simulink model "RealTimeSimulation"  (R2024b)
settings: Solver=ode45  StartTime=0.0  StopTime=20  FixedStep=0.001  RelTol=1e-3
InitFcn:
  | Init
values from neighbouring files (symbols this model uses):
  Beq = 1.223604206496999e-06    (= 1.2236042065e-06)    [DesignPart567.m]    (also in DesignPart9Sine.m; DesignPart9Step.m; Init.m; Real_time_parameter_estimation.m = (data.Beq_hat_pos + data.Beq_hat_neg)/2)
  degs2rpm = 60/360    (= 0.166666666667)    [Init.m]
  delta_est = 1/sqrt(2)    [DesignPart9Step.m]    (also in Init.m)
  Kd = Kp * Td    [Init.m]
  Ki = Kp / Ti    [Init.m]
  Kp = deltak * cos(deltaphi)    [Init.m]
  rpm2degs = 360/60    (= 6)    [Init.m]
  rpm2rads = 2*pi/60    (= 0.10471975512)    [Init.m]
  tau_sf = (abs(data.tau_sf_pos)+abs(data.tau_sf_neg))/2    [Real_time_parameter_estimation.m]    (also in real-time-estimation.mat = 0.0046178193958)
  tl = 1/(3*wgc)    [Init.m]
  wc = 2*pi*50    (= 314.159265359)    [DesignPart9Step.m]    (also in Init.m; State_space_1324.m)
undefined symbols (not defined in the file or in its folder): gbox, mot, sens
libraries: simulink x2
settings Model: Creator=Banaan  LastModifiedBy=lucag

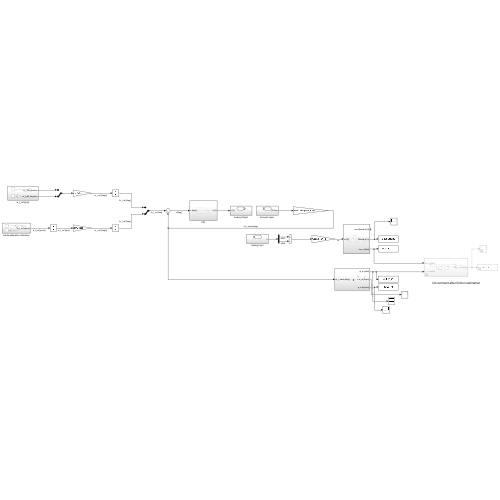
[thumbnail: Simulink's stored preview of the top-level diagram]
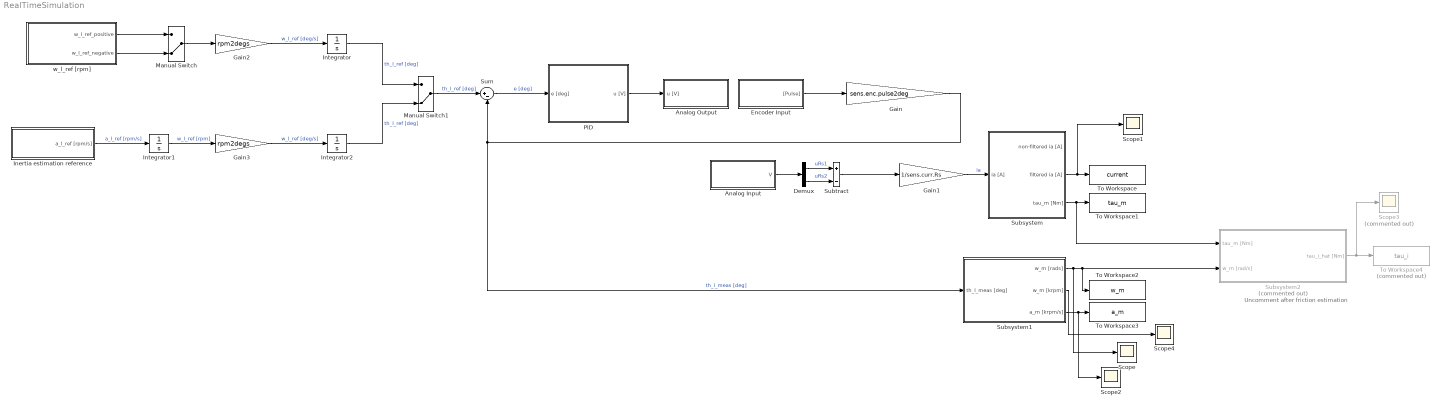
== system RealTimeSimulation ==
  note: Uncomment after friction estimation
  Analog Input : Subsystem
  Analog Output : Subsystem
  Demux : Demux  Outputs=2
  Encoder Input : Subsystem
  Gain : Gain  Gain=sens.enc.pulse2deg
  Gain1 : Gain  Gain=1/sens.curr.Rs
  Gain2 : Gain  Gain=rpm2degs
  Gain3 : Gain  Gain=rpm2degs
  Inertia estimation reference : Subsystem
  Integrator : Integrator
  Integrator1 : Integrator
  Integrator2 : Integrator
  Manual Switch : ManualSwitch  CurrentSetting=0
  Manual Switch1 : ManualSwitch  CurrentSetting=0
  PID : Subsystem
  Scope{,1..2,4} (4 alike) : Scope
  Scope3 : Scope  Commented=on
  Subsystem : Subsystem
  Subsystem1 : Subsystem
  Subsystem2 : Subsystem  Commented=on
  Subtract : Sum  Inputs=+-
  Sum : Sum  Inputs=|+-
  To Workspace : ToWorkspace  VariableName=current  SaveFormat=Structure With Time  SampleTime=-1
  To Workspace1 : ToWorkspace  VariableName=tau_m  SaveFormat=Structure With Time  SampleTime=-1
  To Workspace2 : ToWorkspace  VariableName=w_m  SaveFormat=Structure With Time  SampleTime=-1
  To Workspace3 : ToWorkspace  VariableName=a_m  SaveFormat=Structure With Time  SampleTime=-1
  To Workspace4 : ToWorkspace  Commented=on  VariableName=tau_i  SaveFormat=Structure With Time  SampleTime=-1
  w_l_ref [rpm] : Subsystem
  wires:
  Gain/1 -> Subsystem1/1(th_l_meas [deg]), Sum/2  "th_l_meas [deg]"
  Sum/1 -> PID/1(e [deg])  "e [deg]"
  Manual Switch1/1 -> Sum/1  "th_l_ref [deg]"
  Analog Input/1(V) -> Demux/1
  Demux/1 -> Subtract/1  "uRs1"
  Demux/2 -> Subtract/2  "uRs2"
  Gain1/1 -> Subsystem/1(ia [A])  "ia"
  Subsystem/2(filtered ia [A]) -> Scope1/1, To Workspace/1
  Subsystem/3(tau_m [Nm]) -> Subsystem2/1(tau_m [Nm]), To Workspace1/1
  Gain2/1 -> Integrator/1  "w_l_ref [deg/s]"
  Integrator/1 -> Manual Switch1/1  "th_l_ref [deg]"
  Gain3/1 -> Integrator2/1  "w_l_ref [deg/s]"
  Inertia estimation reference/1(a_l_ref [rpm/s]) -> Integrator1/1  "a_l_ref [rpm/s]"
  Integrator1/1 -> Gain3/1  "w_l_ref [rpm]"
  Integrator2/1 -> Manual Switch1/2  "th_l_ref [deg]"
  Manual Switch/1 -> Gain2/1
  w_l_ref [rpm]/1(w_l_ref_positive) -> Manual Switch/1
  w_l_ref [rpm]/2(w_l_ref_negative) -> Manual Switch/2
  Subsystem1/1(w_m [rads]) -> Subsystem2/2(w_m [rad/s]), To Workspace2/1, Scope/1
  Subsystem1/3(a_m [krpm/s]) -> Scope2/1, To Workspace3/1
  Subsystem2/1(tau_i_hat [Nm]) -> Scope3/1, To Workspace4/1
  Subsystem1/2(w_m [krpm]) -> Scope4/1
  PID/1(u [V]) -> Analog Output/1(u [V])
  Encoder Input/1("[Pulse]") -> Gain/1
  Subtract/1 -> Gain1/1

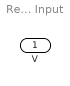
== system RealTimeSimulation/Analog Input ==
  V : Outport

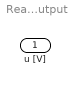
== system RealTimeSimulation/Analog Output ==
  u [V] : Inport

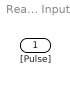
== system RealTimeSimulation/Encoder Input ==
  "[Pulse]" : Outport

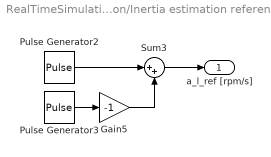
== system RealTimeSimulation/Inertia estimation reference ==
  Gain5 : Gain  Gain=-1
  Pulse Generator2 : DiscretePulseGenerator  PulseType=Time based  Amplitude=450  PulseWidth=50
  Pulse Generator3 : DiscretePulseGenerator  PulseType=Time based  Amplitude=450  PulseWidth=50  PhaseDelay=1
  Sum3 : Sum  Inputs=|++
  a_l_ref [rpm/s] : Outport
  wires:
  Pulse Generator3/1 -> Gain5/1
  Pulse Generator2/1 -> Sum3/1
  Gain5/1 -> Sum3/2
  Sum3/1 -> a_l_ref [rpm/s]/1

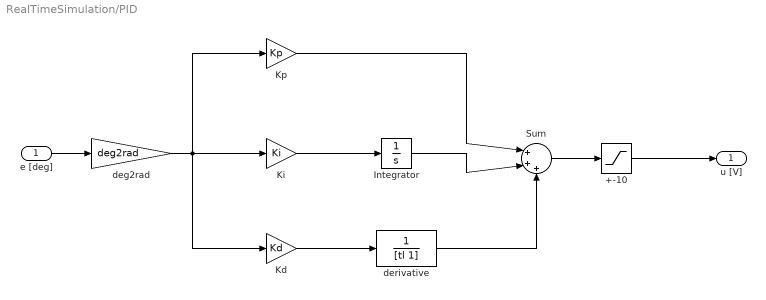
== system RealTimeSimulation/PID ==
  e [deg] : Inport
  +-10 : Saturate  UpperLimit=10  LowerLimit=-10
  Integrator : Integrator
  Kd : Gain  Gain=Kd
  Ki : Gain  Gain=Ki
  Kp : Gain  Gain=Kp
  Sum : Sum  Inputs=|+++
  deg2rad : Gain  Gain=deg2rad
  derivative : TransferFcn  Denominator=[tl 1]
  u [V] : Outport
  wires:
  e [deg]/1 -> deg2rad/1
  deg2rad/1 -> Kd/1, Kp/1, Ki/1
  Ki/1 -> Integrator/1
  Kp/1 -> Sum/1
  Integrator/1 -> Sum/2
  Kd/1 -> derivative/1
  derivative/1 -> Sum/3
  Sum/1 -> +-10/1
  +-10/1 -> u [V]/1

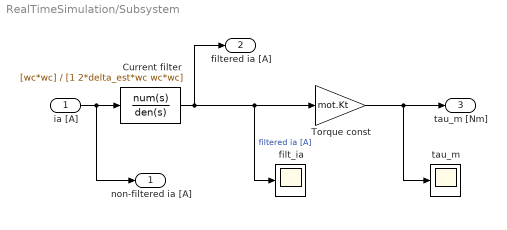
== system RealTimeSimulation/Subsystem ==
  ia [A] : Inport
  " Current filter" : TransferFcn  Numerator=[wc*wc]  Denominator=[1 2*delta_est*wc wc*wc]
  Torque const : Gain  Gain=mot.Kt
  filt_ia : Scope
  tau_m : Scope
  non-filtered ia [A] : Outport
  filtered ia [A] : Outport  Port=2
  tau_m [Nm] : Outport  Port=3
  wires:
  " Current filter"/1 -> filtered ia [A]/1, filt_ia/1, Torque const/1  "filtered ia [A]"
  Torque const/1 -> tau_m [Nm]/1, tau_m/1
  ia [A]/1 -> non-filtered ia [A]/1, " Current filter"/1

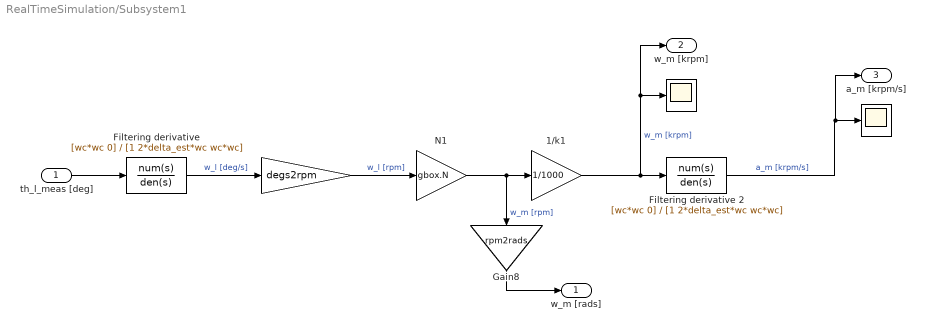
== system RealTimeSimulation/Subsystem1 ==
  th_l_meas [deg] : Inport
  " " : Gain  Gain=degs2rpm
  "  " : Scope
  "    " : Scope
  1/k1 : Gain  Gain=1/1000
  Filtering derivative : TransferFcn  Numerator=[wc*wc 0]  Denominator=[1 2*delta_est*wc wc*wc]
  Filtering derivative 2 : TransferFcn  Numerator=[wc*wc 0]  Denominator=[1 2*delta_est*wc wc*wc]
  Gain8 : Gain  Gain=rpm2rads
  N1 : Gain  Gain=gbox.N
  w_m [rads] : Outport
  w_m [krpm] : Outport  Port=2
  a_m [krpm/s] : Outport  Port=3
  wires:
  N1/1 -> Gain8/1, 1/k1/1  "w_m [rpm]"
  1/k1/1 -> "  "/1, w_m [krpm]/1, Filtering derivative 2/1  "w_m [krpm]"
  Gain8/1 -> w_m [rads]/1
  Filtering derivative/1 -> " "/1  "w_l [deg/s]"
  Filtering derivative 2/1 -> a_m [krpm/s]/1, "    "/1  "a_m [krpm/s]"
  " "/1 -> N1/1  "w_l [rpm]"
  th_l_meas [deg]/1 -> Filtering derivative/1

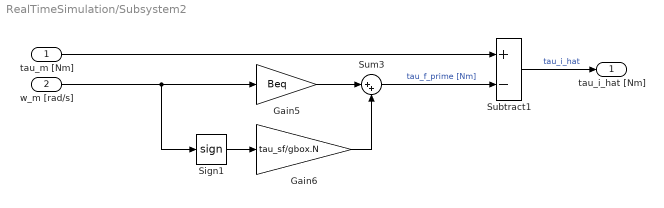
== system RealTimeSimulation/Subsystem2 ==
  tau_m [Nm] : Inport
  w_m [rad/s] : Inport  Port=2
  Gain5 : Gain  Gain=Beq
  Gain6 : Gain  Gain=tau_sf/gbox.N
  Sign1 : Signum  ZeroCross=off
  Subtract1 : Sum  Inputs=+-
  Sum3 : Sum  Inputs=|++
  tau_i_hat [Nm] : Outport
  wires:
  Subtract1/1 -> tau_i_hat [Nm]/1  "tau_i_hat"
  tau_m [Nm]/1 -> Subtract1/1
  Gain5/1 -> Sum3/1
  Sum3/1 -> Subtract1/2  "tau_f_prime [Nm]"
  Sign1/1 -> Gain6/1
  Gain6/1 -> Sum3/2
  w_m [rad/s]/1 -> Sign1/1, Gain5/1

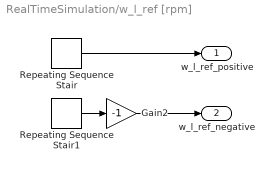
== system RealTimeSimulation/w_l_ref [rpm] ==
  Gain2 : Gain  Gain=-1
  Repeating Sequence Stair : simulink/Sources/Repeating Sequence Stair  OutValues=[50 100 150 200 250 300 350 400 450 450].'  tsamp=5  OutMin=[]  OutMax=[]  OutDataTypeStr=double  OutputDataTypeScalingMode=double  OutDataType=fixdt(0,8)  ConRadixGroup=Best Precision: Vector-wise  OutScaling=2^-12
  Repeating Sequence Stair1 : simulink/Sources/Repeating Sequence Stair  OutValues=[50 100 150 200 250 300 350 400 450 450].'  tsamp=5  OutMin=[]  OutMax=[]  OutDataTypeStr=double  OutputDataTypeScalingMode=double  OutDataType=fixdt(0,8)  ConRadixGroup=Best Precision: Vector-wise  OutScaling=2^-12
  w_l_ref_positive : Outport
  w_l_ref_negative : Outport  Port=2
  wires:
  Repeating Sequence Stair1/1 -> Gain2/1
  Gain2/1 -> w_l_ref_negative/1
  Repeating Sequence Stair/1 -> w_l_ref_positive/1
